simulink model "Simulink_Model"  (R2016b)
settings: Solver=VariableStepAuto  StartTime=0.0  StopTime=40  RelTol=1e-3
undefined symbols (not defined in the file): T
settings Model: Creator=Milan Sas  LastModifiedBy=Milan Sas

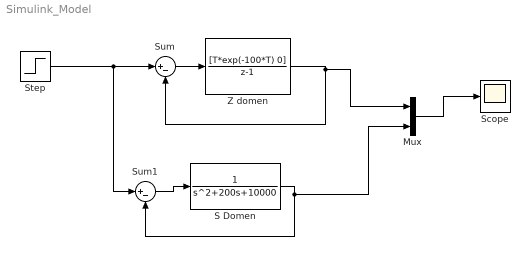
== system Simulink_Model ==
  Mux : Mux  Inputs=2
  S Domen : TransferFcn  Denominator=[1 200 10000]
  Scope : Scope
  Step : Step  SampleTime=0
  Sum : Sum  Inputs=|+-
  Sum1 : Sum  Inputs=|+-
  Z domen : DiscreteTransferFcn  Numerator=[T*exp(-100*T) 0]  Denominator=[1 -1]  SampleTime=T
  wires:
  Step/1 -> Sum1/1, Sum/1
  Sum/1 -> Z domen/1
  Z domen/1 -> Mux/1, Sum/2
  Sum1/1 -> S Domen/1
  S Domen/1 -> Mux/2, Sum1/2
  Mux/1 -> Scope/1
